simulink model "jointTorqueCtrl_reachPos_minJerk_sync"  (Simulink 8.0)
settings: Solver=FixedStepDiscrete  StartTime=0.0  StopTime=Inf  FixedStep=Ts  RelTol=1e-3
undefined symbols (not defined in the file or in its folder): displayMask, dqErr, dqiRef, GRAV_COMP, Kd, KdOnOff, Kp, KpOnOff, MOnOff, qErr, qjDes, refMask, refMaskGravComp, ROBOT_DOF, Ts
libraries: WBCLibrary x17
settings Model: Creator=nunoguedelha  LastModifiedBy=nunoguedelha

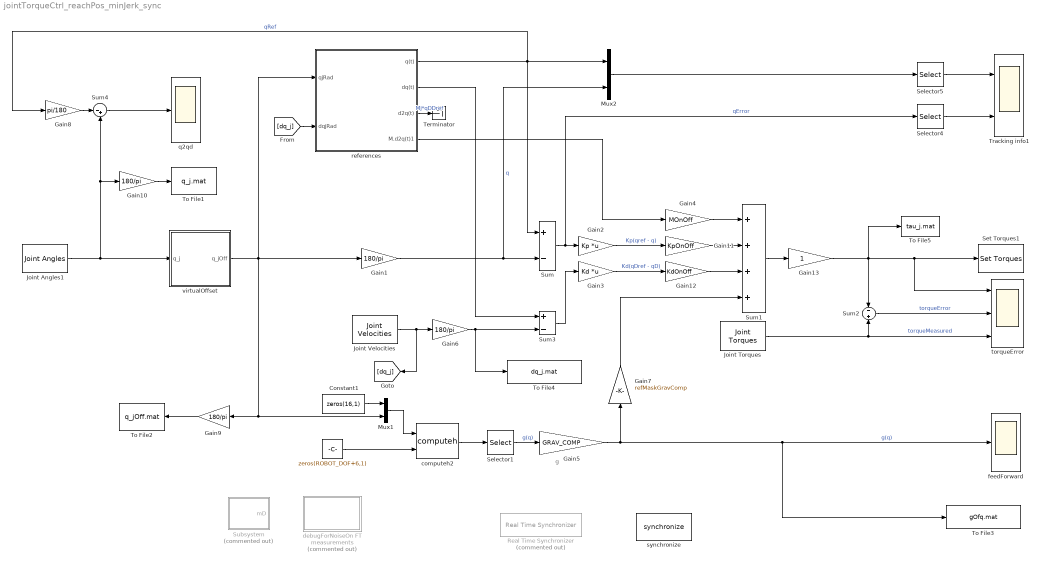
== system jointTorqueCtrl_reachPos_minJerk_sync ==
  note: g
  " " : Constant  Tag=bla  Value=zeros(ROBOT_DOF+6,1)  SampleTime=-1
  Constant1 : Constant  Value=zeros(16,1)  SampleTime=-1
  Gain{1,6,9..10} (4 alike) : Gain  Gain=180/pi
  Gain11 : Gain  Gain=KpOnOff
  Gain12 : Gain  Gain=KdOnOff
  Gain13 : Gain
  Gain2 : Gain  Gain=Kp  Multiplication=Matrix(K*u)
  Gain3 : Gain  Gain=Kd  Multiplication=Matrix(K*u)
  Gain4 : Gain  Gain=MOnOff
  Gain5 : Gain  Gain=GRAV_COMP
  Gain7 : Gain  Gain=refMaskGravComp
  Gain8 : Gain  Gain=pi/180
  Joint Angles1 : WBCLibrary/wholeBodyStates/Joint Angles  robotName=robotName  localName=localName
  Joint Torques : WBCLibrary/wholeBodyStates/Joint Torques  robotName=robotName  localName=localName
  Joint Velocities : WBCLibrary/wholeBodyStates/Joint Velocities  robotName=robotName  localName=localName
  Mux1 : Mux  Inputs=2
  Mux2 : Mux  Inputs=2
  Real Time Synchronizer : WBCLibrary/Utilities/Real Time Synchronizer  Priority=-10  Commented=on  threadPeriod=Ts
  Selector1 : Selector  InputPortWidth=ROBOT_DOF+6  IndexOptions=Index vector (dialog)  Indices=[7:ROBOT_DOF+6]  OutputSizes=1
  Selector4 : Selector  InputPortWidth=ROBOT_DOF  IndexOptions=Index vector (dialog)  Indices=[displayMask]  OutputSizes=1
  Selector5 : Selector  InputPortWidth=2*ROBOT_DOF  IndexOptions=Index vector (dialog)  Indices=[displayMask ROBOT_DOF+displayMask]  OutputSizes=1
  Set Torques1 : WBCLibrary/wholeBodyActuators/Set Torques  val=6  robotName=robotName  localName=localName
  Subsystem : Subsystem  Commented=on
  Sum : Sum  Inputs=+-
  Sum1 : Sum  Inputs=++++
  Sum2 : Sum  Inputs=-|+
  Sum3 : Sum  Inputs=+-
  Sum4 : Sum  Inputs=|-+
  Terminator : Terminator
  To File1 : ToFile  Filename=q_j.mat  SaveFormat=Timeseries
  To File2 : ToFile  Filename=q_jOff.mat  SaveFormat=Timeseries
  To File3 : ToFile  Filename=gOfq.mat  SaveFormat=Timeseries
  To File4 : ToFile  Filename=dq_j.mat  SaveFormat=Timeseries
  To File5 : ToFile  Filename=tau_j.mat  SaveFormat=Timeseries
  Tracking info1 : Scope  NumInputPorts=2
      settings: ShowLegends=on  TimeRange=20  YMin=-60~-5  YMax=80~5  SaveName=ScopeData6
  computeh2 : WBCLibrary/wholeBodyModel/Dynamics/computeh  val=7  robotname=robotName  localname=localName
  debugForNoiseOn FT measurements : Subsystem  Commented=on
  feedForward : Scope
      settings: ShowLegends=on  TimeRange=70  YMin=-1  YMax=1
  q2qd : Scope
      settings: ShowLegends=on  TimeRange=20  YMin=-60  YMax=80  SaveName=ScopeData7
  references : Subsystem
  synchronize : WBCLibrary/Utilities/synchronize  rate=0.010  scaleFactor=1
  torqueError : Scope  NumInputPorts=3
      settings: ShowLegends=on  TimeRange=20  YMin=-3~-2~-2  YMax=3~3~2
  virtualOffset : MATLAB Function  TreatAsAtomicUnit=on
  wires:
  Gain1/1 -> Mux2/2, Sum/2  "q"
  Sum/1 -> Selector4/1, Gain2/1  "qError"
  Gain2/1 -> Gain11/1  "Kp(qref - q)"
  Joint Velocities/1 -> [dq_j], Gain6/1
  Gain3/1 -> Gain12/1  "Kd(qDref - qD)"
  computeh2/1 -> Selector1/1
  Mux1/1 -> computeh2/1
  Constant1/1 -> Mux1/1
  Selector1/1 -> Gain5/1  "g(q)"
  Joint Torques/1 -> torqueError/3, Sum2/2  "torqueMeasured"
  Sum2/1 -> torqueError/2  "torqueError"
  Gain5/1 -> feedForward/1, To File3/1, Gain7/1  "g(q)"
  references/1(q(t)) -> Sum/1, Mux2/1, Gain8/1  "qRef"
  Gain6/1 -> To File4/1, Sum3/2
  Sum3/1 -> Gain3/1
  references/2(dq(t)) -> Sum3/1
  " "/1 -> computeh2/2
  Sum1/1 -> Gain13/1
  references/3(d2q(t)) -> Terminator/1  "Mj*qDDref"
  Selector4/1 -> Tracking info1/2
  Gain7/1 -> Sum1/4
  virtualOffset/1(q_jOff) -> Gain1/1, references/1(qjRad), Mux1/2, Gain9/1
  Sum4/1 -> q2qd/1
  Gain8/1 -> Sum4/1
  Mux2/1 -> Selector5/1
  Selector5/1 -> Tracking info1/1
  references/4(M.d2q(t)1) -> Gain4/1
  Joint Angles1/1 -> virtualOffset/1(q_j), Gain10/1, Sum4/2
  Gain10/1 -> To File1/1
  Gain9/1 -> To File2/1
  [dq_j] -> references/2(dqjRad)
  Gain4/1 -> Sum1/1
  Gain11/1 -> Sum1/2
  Gain12/1 -> Sum1/3
  Gain13/1 -> To File5/1, Sum2/1, torqueError/1, Set Torques1/1

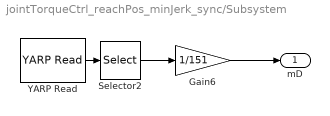
== system jointTorqueCtrl_reachPos_minJerk_sync/Subsystem ==
  Gain6 : Gain  Gain=1/151
  Selector2 : Selector  InputPortWidth=6  IndexOptions=Index vector (dialog)  Indices=[1]  OutputSizes=1
  YARP Read : WBCLibrary/Utilities/YARP Read  portName='/controlBoardDumper/right_leg/getMotorEncoderSpeeds'  signalSize=6  blocking=off  timestamp=off  autoconnect=on  errorOnConnection=off
  mD : Outport
  wires:
  YARP Read/1 -> Selector2/1
  Selector2/1 -> Gain6/1
  Gain6/1 -> mD/1

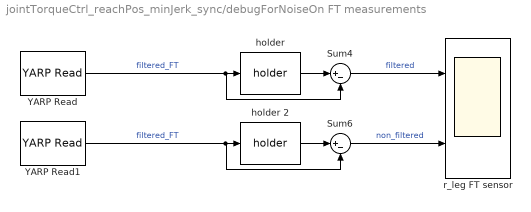
== system jointTorqueCtrl_reachPos_minJerk_sync/debugForNoiseOn FT measurements ==
  Sum4 : Sum  Inputs=|+-
  Sum6 : Sum  Inputs=|+-
  YARP Read : WBCLibrary/Utilities/YARP Read  portName='/wholeBodyDynamicsTree/filtered/r_leg_ft_sensor:o'  signalSize=6  blocking=off  timestamp=off  autoconnect=on  errorOnConnection=off
  YARP Read1 : WBCLibrary/Utilities/YARP Read  portName='/icub/right_leg/analog:o'  signalSize=6  blocking=off  timestamp=off  autoconnect=on  errorOnConnection=off
  "holder " : WBCLibrary/Utilities/holder 
  holder 2 : WBCLibrary/Utilities/holder 
  r_leg FT sensor : Scope  NumInputPorts=2
      settings: ShowLegends=on  TimeRange=10  YMin=-10~-15  YMax=15~20  SaveName=ScopeData5
  wires:
  "holder "/1 -> Sum4/1
  YARP Read/1 -> Sum4/2, "holder "/1  "filtered_FT"
  Sum6/1 -> r_leg FT sensor/2  "non_filtered"
  YARP Read1/1 -> Sum6/2, holder 2/1  "filtered_FT"
  holder 2/1 -> Sum6/1
  Sum4/1 -> r_leg FT sensor/1  "filtered"

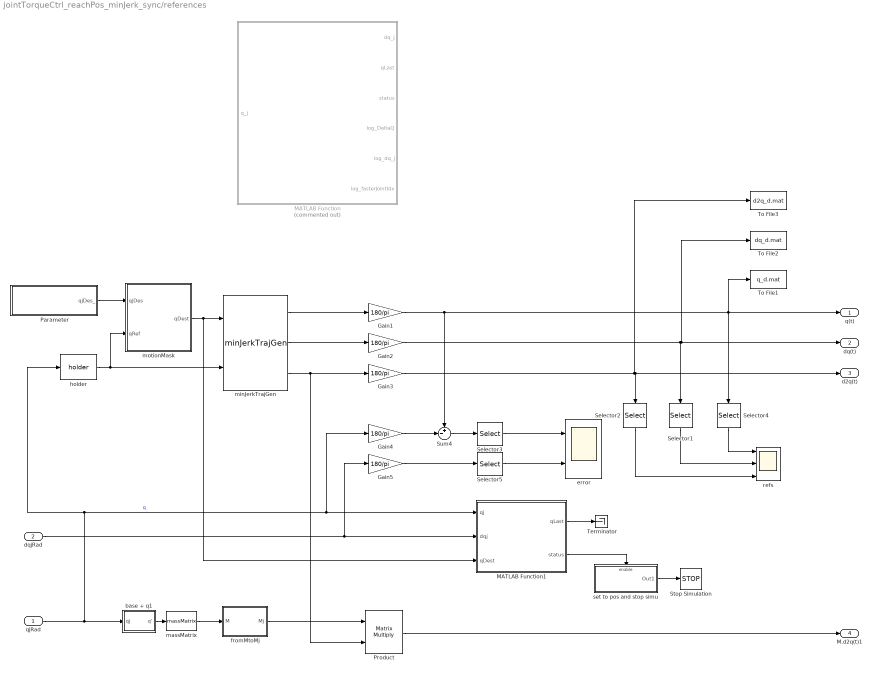
== system jointTorqueCtrl_reachPos_minJerk_sync/references ==
  qjRad : Inport
  dqjRad : Inport  Port=2
  Gain{1..5} (5 alike) : Gain  Gain=180/pi
  MATLAB Function : MATLAB Function  Commented=on  TreatAsAtomicUnit=on
  MATLAB Function1 : MATLAB Function  TreatAsAtomicUnit=on
  Parameter : MATLAB Function  TreatAsAtomicUnit=on
  Product : Product  Multiplication=Matrix(*)
  Selector{1..5} (5 alike) : Selector  InputPortWidth=ROBOT_DOF  IndexOptions=Index vector (dialog)  Indices=[displayMask]  OutputSizes=1
  Stop Simulation : Stop
  Sum4 : Sum  Inputs=+-|
  Terminator : Terminator
  To File1 : ToFile  Filename=q_d.mat  SaveFormat=Timeseries
  To File2 : ToFile  Filename=dq_d.mat  SaveFormat=Timeseries
  To File3 : ToFile  Filename=d2q_d.mat  SaveFormat=Timeseries
  base + q1 : Subsystem
  error : Scope  NumInputPorts=2
      settings: ShowLegends=on  TimeRange=70  YMin=-17.5~-0.25  YMax=17.5~0.2  SaveName=ScopeData3
  fromMtoMj : MATLAB Function  TreatAsAtomicUnit=on
  "holder " : WBCLibrary/Utilities/holder 
  massMatrix : WBCLibrary/wholeBodyModel/Dynamics/massMatrix  val=8  robotname=robotName  localname=localName
  minJerkTrajGen : WBCLibrary/Utilities/minJerkTrajGen  dim=ROBOT_DOF  Ts=Ts  Tt=Tt
  motionMask : MATLAB Function  TreatAsAtomicUnit=on
  refs : Scope  NumInputPorts=3
      settings: ShowLegends=on  TimeRange=70  YMin=-80~-10~-5  YMax=110~2~17.5  SaveName=ScopeData2
  set to pos and stop simu : Subsystem  TreatAsAtomicUnit=on
  q(t) : Outport
  dq(t) : Outport  Port=2
  d2q(t) : Outport  Port=3
  M.d2q(t)1 : Outport  Port=4
  wires:
  minJerkTrajGen/1 -> Gain1/1
  minJerkTrajGen/2 -> Gain2/1
  base + q1/1(q') -> massMatrix/1
  Product/1 -> M.d2q(t)1/1
  massMatrix/1 -> fromMtoMj/1(M)
  fromMtoMj/1(Mj) -> Product/1
  minJerkTrajGen/3 -> Gain3/1, Product/2
  qjRad/1 -> base + q1/1(qj), Gain4/1, MATLAB Function1/1(qj), "holder "/1  "q"
  "holder "/1 -> minJerkTrajGen/2, motionMask/2(qRef)
  motionMask/1(qDest) -> MATLAB Function1/3(qDest), minJerkTrajGen/1
  Gain1/1 -> Sum4/1, To File1/1, Selector4/1, q(t)/1
  Gain2/1 -> dq(t)/1, To File2/1, Selector1/1
  Gain3/1 -> Selector2/1, d2q(t)/1, To File3/1
  Parameter/1(qjDes_) -> motionMask/1(qjDes)
  MATLAB Function1/1(qLast) -> Terminator/1
  MATLAB Function1/2(status) -> set to pos and stop simu/Enable
  dqjRad/1 -> MATLAB Function1/2(dqj), Gain5/1
  Selector4/1 -> refs/1
  Selector1/1 -> refs/2
  Selector2/1 -> refs/3
  Gain4/1 -> Sum4/2
  Sum4/1 -> Selector3/1
  Selector3/1 -> error/1
  Selector5/1 -> error/2
  Gain5/1 -> Selector5/1
  set to pos and stop simu/1(Out1) -> Stop Simulation/1

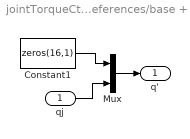
== system jointTorqueCtrl_reachPos_minJerk_sync/references/base + q1 ==
  qj : Inport
  Constant1 : Constant  Value=zeros(16,1)
  Mux : Mux  Inputs=2
  q' : Outport
  wires:
  Mux/1 -> q'/1
  qj/1 -> Mux/2
  Constant1/1 -> Mux/1

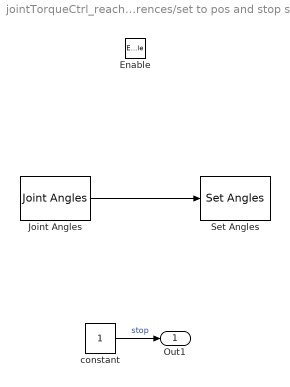
== system jointTorqueCtrl_reachPos_minJerk_sync/references/set to pos and stop simu ==
  Enable : EnablePort
  Joint Angles : WBCLibrary/wholeBodyStates/Joint Angles  robotName=robotName  localName=localName
  Set Angles : WBCLibrary/wholeBodyActuators/Set Angles  val=5  robotName=robotName  localName=localName
  constant : Constant  SampleTime=-1
  Out1 : Outport  OutputWhenDisabled=reset  InitialOutput=0
  wires:
  Joint Angles/1 -> Set Angles/1
  constant/1 -> Out1/1  "stop"

== matlab function references/MATLAB Function ==
  data: dq_j output double; qjDes parameter double; dqiRef parameter double; q_j input double; ROBOT_DOF parameter double; qErr parameter double; Ts parameter double; qLast output double; status output double; log_DeltaQ output double; log_dq_j output double; log_fasterJointIdx output double
function [dq_j, qLast, status, log_DeltaQ, log_dq_j, log_fasterJointIdx]  = checkStopCond(qjDes, dqiRef, q_j, ROBOT_DOF, qErr, Ts)
%#codegen

% define the maximum speed (in degrees) of the reference revolute single joint
% (single DOF). This is done manually:
% joints rotation speed is considered constant, so we only get centripete 
% acceleration . $|a_n| = \frac{v^2}{R} = R dq^2$
% => $dqiRef = \sqrt{\frac{|a_n|}{R}}$
% As a_n max should not exceed 1/10 g,
% $dqiRef = \sqrt{\frac{1}{R}} ~ sqrt(1/0.4) ~ 1.5 rad.s^{-1} = 85 degs.s^{-1}$ for $g ~
% 10m.s^{-2}$.
% Let's have a margin and define $45 deg.s^{-1}$ (signed value)
persistent fasterJointIdx;
persistent last_dq_j;
persistent last_deltaQ;
persistent stopMotionVec;
persistent state;

dq_j = zeros(ROBOT_DOF,1);

%% handle state
if isempty(state)
    state = 0;
end

% update positions relative to the destination
DeltaQ = qjDes - q_j;

% Fill static variables
if isempty(last_deltaQ)
    last_deltaQ = DeltaQ;
end

if isempty(stopMotionVec)
    stopMotionVec = ones(ROBOT_DOF,1);
end

if isempty(fasterJointIdx)
    % Select joint for which rotation will have the highest speed.
    % This shall be the high boundary speed for all joints. We shall set this
    % boundary to the maximum speed 'dqiRef' required for neglecting the angular
    % and linear acceleration to be measured by the sensors, w.r.t. the gravity
    % measurements.
    [~,idx_of_max] = max(abs(DeltaQ));
    fasterJointIdx = uint8(idx_of_max); % convert to uint8
end

if isempty(last_dq_j)
    last_dq_j = zeros(ROBOT_DOF,1);
end


if state == 0
    %% Program joint velocity for current timeslot

    % If angles are small, avoid computing dq_j, just use same velocities for
    % all joints.
    if abs(DeltaQ(fasterJointIdx))>(5*pi/180)
        dq_j = DeltaQ*(dqiRef/abs(DeltaQ(fasterJointIdx)));
        last_dq_j = dq_j;
    else
        dq_j = last_dq_j;
    end
    
    % We shall stop as soon as the joint closest to its respective end position
    % reaches the end position vicinity (d<0.1 deg) or overshoots.
    % Considering that the velocity or position tracking accuracy is not perfect, 
    % we should monitor each joint independently.
    for i = 1:ROBOT_DOF
    if abs(DeltaQ(i))<(dqiRef*10*Ts) ... % proximity
            || last_deltaQ(i)*DeltaQ(i)<0 % overshoot
        % mark respective joint for stopping
        stopMotionVec(i) = 0;
    end
    end
    
    % Stop the joints that reached destination
    dq_j = dq_j.*stopMotionVec;
    
    if any(dq_j)
        state = 0;
        last_deltaQ = DeltaQ;
    else
        % final configuration reached
        state = 1;
    end
end

% save last position
qLast = q_j;
% output state
status = state;

%log DeltaQ and dq_j
log_DeltaQ = DeltaQ;
log_dq_j = dq_j;
log_fasterJointIdx = fasterJointIdx;

% we would clear the static variables here but 'clear' is not supported
% in generated code

end

== matlab function references/fromMtoMj ==
  data: M input double; Mj output double
function Mj = fromMtoMj(M)
%#codegen

Mj = M(7:end,7:end);

== matlab function references/motionMask ==
  data: qjDes input double; qRef input double; refMask parameter double; qDest output double; ROBOT_DOF parameter double
function qDest = motionMask(qjDes,qRef,refMask,ROBOT_DOF)
%#codegen

% Target position
qDest = qjDes.*refMask + qRef.*(ones(ROBOT_DOF,1)-refMask);

== matlab function references/Parameter ==
  data: qjDes parameter double; qjDes_ output double
function qjDes_ = getParameter(qjDes)
%#codegen
qjDes_ = qjDes;

== matlab function virtualOffset ==
  data: q_j input double; q_jOff output double; randOffsets parameter double
function q_jOff = refMaskGravComp(q_j,randOffsets)
%#codegen


q_jOff = q_j + randOffsets;

== matlab function references/MATLAB Function1 ==
  data: qj input double; qLast output double; status output double; dqj input double; qDest input double; qErr parameter double; dqErr parameter double
function [qLast,status] = stopCondition(qj,dqj,qDest,qErr,dqErr)
%#codegen

if (norm(qj-qDest,2)<qErr && norm(dqj,2)<dqErr)
    status = 1;
else
    status = 0;
end

qLast = qj;
